simulink model "vector_rotation"  (R2018a)
settings: Solver=VariableStepAuto  StartTime=0.0  StopTime=10.0  RelTol=1e-3
settings Model: Creator=Rafael  LastModifiedBy=Rafael
settings DataIOCC: SaveOutput=off  SaveTime=off

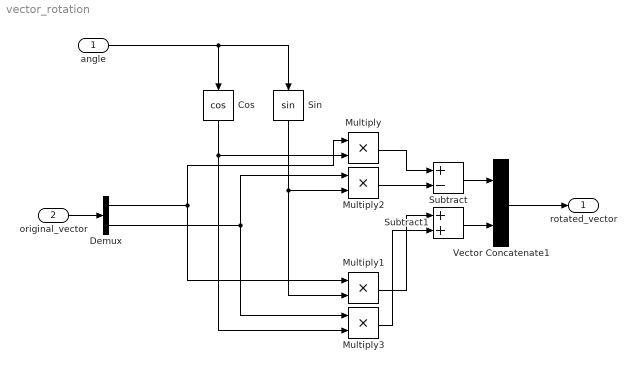
== system vector_rotation ==
  angle : Inport  OutDataTypeStr=double  PortDimensions=1  SampleTime=0
  original_vector : Inport  Port=2  OutDataTypeStr=double  PortDimensions=2
  Cos : Trigonometry  Operator=cos
  Demux : Demux  Outputs=2
  Multiply{,1..3} (4 alike) : Product
  Sin : Trigonometry
  Subtract : Sum  Inputs=+-
  Subtract1 : Sum
  Vector Concatenate1 : Concatenate
  "rotated_vector " : Outport  OutDataTypeStr=double  PortDimensions=2  SampleTime=0
  wires:
  Multiply3/1 -> Subtract1/2
  Multiply1/1 -> Subtract1/1
  Multiply/1 -> Subtract/1
  Demux/2 -> Multiply2/1, Multiply3/1
  Subtract1/1 -> Vector Concatenate1/2
  Cos/1 -> Multiply/2, Multiply3/2
  Sin/1 -> Multiply2/2, Multiply1/2
  angle/1 -> Sin/1, Cos/1
  Demux/1 -> Multiply1/1, Multiply/1
  Vector Concatenate1/1 -> "rotated_vector "/1
  Subtract/1 -> Vector Concatenate1/1
  Multiply2/1 -> Subtract/2
  original_vector/1 -> Demux/1
